simulink model "sf_eventfcn"  (R2017b)
settings: Solver=ode45  StartTime=0.0  StopTime=30  MaxStep=1  RelTol=1e-3  EnableMultiTasking=on
settings Model: FPTRunName=Active  ExtModeAutoUpdateStatusClock=off  Creator=The MathWorks, Inc.  LastModifiedBy=The MathWorks, Inc.
settings DataIOCC: LimitDataPoints=on  SaveFormat=Array  SignalLoggingName=sigsOut
settings OptimizationCC: BooleanDataType=off  ExpressionDepthLimit=2147483647  InitFltsAndDblsToZero=on  EfficientMapNaN2IntZero=off  LifeSpan=inf
settings DebuggingCC: SaveWithParameterizedLinksMsg=none  UnderspecifiedInitializationDetection=Classic  MergeDetectMultiDrivingBlocksExec=none  SignalResolutionControl=TryResolveAllWithWarning  MultiTaskDSMMsg=warning  MultiTaskCondExecSysMsg=none  FcnCallInpInsideContextMsg=warning  StateNameClashWarn=warning  StrictBusMsg=None  SFUnexpectedBacktrackingDiag=warning  SFNoUnconditionalDefaultTransitionDiag=warning  SFExecutionAtInitializationDiag=none
settings HardwareCC: ProdBitPerPointer=32  ProdBitPerSizeT=32  ProdBitPerPtrDiffT=32  ProdLargestAtomicFloat=None  ProdIntDivRoundTo=Undefined  ProdEndianess=Unspecified  ProdWordSize=32  ProdHWDeviceType=32-bit Generic  TargetUnknown=on
settings ModelReferenceCC: PropagateSignalLabelsOutOfModel=off
settings SFSimCC: SimParseCustomCode=off
settings CodeAppCC: StateflowObjectComments=on
settings GRTTargetCC: TargetFcnLib=ansi_tfl_tmw.mat  TargetLangStandard=C89/C90 (ANSI)  GeneratePreprocessorConditionals=Disable all  CombineOutputUpdateFcns=off  GRTInterface=on
settings ConfigComp: CovMetricSettings=dcmtr  CovHtmlReporting=on  CovSaveCumulativeToWorkspaceVar=on  CovSaveSingleToWorkspaceVar=on  CovExternalEMLEnable=off  CovSFcnEnable=off

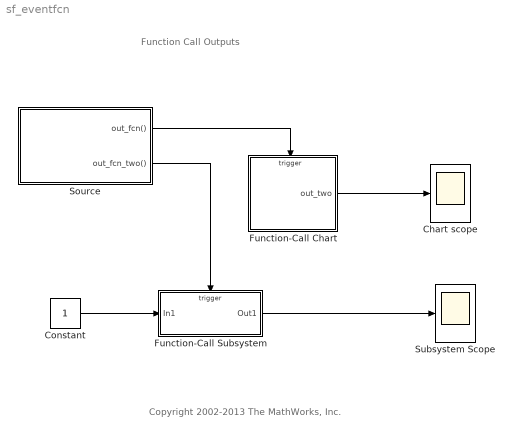
== system sf_eventfcn ==
  note: Function Call Outputs
  note: Copyright 2002-2013 The MathWorks, Inc.
  Chart scope : Scope
  Constant : Constant
  Function-Call Subsystem : Subsystem  TreatAsAtomicUnit=on
  Function-Call Chart : Stateflow chart  TreatAsAtomicUnit=on
  Source : Stateflow chart  TreatAsAtomicUnit=on
  Subsystem Scope : Scope
  wires:
  Source/2(out_fcn_two()) -> Function-Call Subsystem/Trigger
  Source/1(out_fcn()) -> Function-Call Chart/Trigger
  Function-Call Chart/1(out_two) -> Chart scope/1
  Constant/1 -> Function-Call Subsystem/1(In1)
  Function-Call Subsystem/1(Out1) -> Subsystem Scope/1

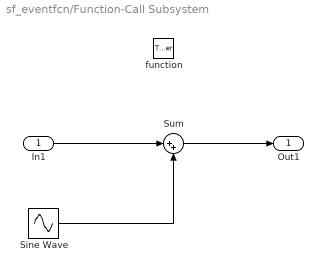
== system sf_eventfcn/Function-Call Subsystem ==
  In1 : Inport
  function : TriggerPort  TriggerType=function-call  VariantControl=(inherit)  ZeroCross=off
  Sine Wave : Sin
  Sum : Sum  Inputs=|++  SaturateOnIntegerOverflow=on  InputSameDT=on  OutDataTypeStr=Inherit: Same as first input
  Out1 : Outport
  wires:
  In1/1 -> Sum/1
  Sum/1 -> Out1/1
  Sine Wave/1 -> Sum/2

== stateflow chart sf_eventfcn/Source ==
  state One [parallel]
    settings: executionOrder=1
    state A
    (default) -> A
    A -> A : after(3,wakeup)/out_fcn;
  state Two [parallel]
    settings: executionOrder=2
    state B
    (default) -> B
    B -> B : after(2,wakeup)/out_fcn_two;
  events: out_fcn output FUNCTION_CALL_EVENT; out_fcn_two output FUNCTION_CALL_EVENT

== stateflow chart sf_eventfcn/Function-Call Chart ==
  state B
    en:out_two=1;
  state A
    en:out_two=0;
  (default) -> A
  A -> B
  B -> A
  data: out_two output double
  events: event input FUNCTION_CALL_EVENT
